simulink model "queueing"  (R2023b)
settings: Solver=VariableStepAuto  StartTime=0.0  StopTime=10.0  RelTol=1e-3
undefined symbols (not defined in the file or in its folder): m, n
settings Model: Creator=miha4  LastModifiedBy=RobotComp.ru
settings RTWCC: GPUComputeCapability=5.0

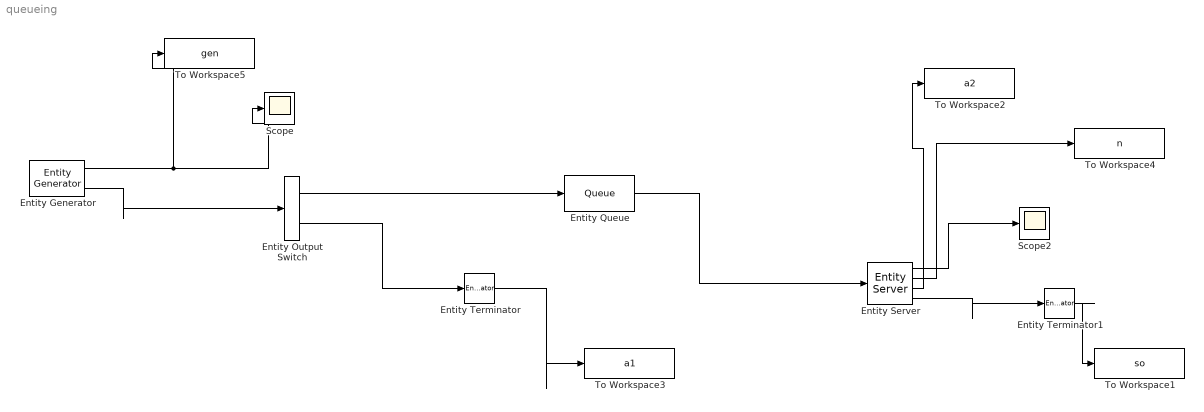
== system queueing ==
  Entity Output Switch : EntityOutputSwitch  InputPortMessageModes=m  OutputPortMessageModes=m,m  SwitchAttributeName=Attribute1
  Entity Generator : EntityGenerator  OutputPortMessageModes=n,m  TimeSource=MATLAB action  IntergenerationTimeAction=|  NumberEntitiesDeparted=on  EntityType=Structured  EntityTypeName=Entity
      | persistent rngInit;
      | if isempty(rngInit)
      |     seed = 12345;
      |     rng(seed);
      |     rngInit = true;
      | end
      | 
      | % Pattern: Exponential distribution
      | mu = 5;
      | dt = -mu * log(1 - rand());
      settings: OutputPortMap=o0,o3
  Entity Queue : Queue  InputPortMessageModes=m  OutputPortMessageModes=m  Capacity=4
  Entity Server : EntityServer  InputPortMessageModes=m  OutputPortMessageModes=n,n,n,m  Capacity=c  ServiceTimeSource=MATLAB action  ServiceTimeValue=500  ServiceTimeAction=|  NumberEntitiesDeparted=on  NumberEntitiesInBlock=on  Utilization=on
      | persistent rngInit;
      | if isempty(rngInit)
      |     seed = 12345;
      |     rng(seed);
      |     rngInit = true;
      | end
      | 
      | % Pattern: Uniform distribution
      | % m: Minimum, M: Maximum
      | m = 2; M = 5;
      | dt = m + (M - m) * rand;
      settings: OutputPortMap=o0,o1,o5,o9
  Entity Terminator : EntityTerminator  InputPortMessageModes=m  NumberEntitiesArrived=on
      settings: OutputPortMap=o0
  Entity Terminator1 : EntityTerminator  InputPortMessageModes=m  NumberEntitiesArrived=on
      settings: OutputPortMap=o0
  Scope : Scope
  Scope2 : Scope
  To Workspace1 : ToWorkspace  VariableName=so  SaveFormat=Timeseries  SampleTime=-1
  To Workspace2 : ToWorkspace  VariableName=a2  SaveFormat=Timeseries  SampleTime=-1
  To Workspace3 : ToWorkspace  VariableName=a1  SaveFormat=Timeseries  SampleTime=-1
  To Workspace4 : ToWorkspace  VariableName=n  SaveFormat=Timeseries  SampleTime=-1
  To Workspace5 : ToWorkspace  VariableName=gen  SaveFormat=Timeseries  SampleTime=-1
  wires:
  Entity Output Switch/1 -> Entity Queue/1
  Entity Server/3 -> To Workspace2/1
  Entity Output Switch/2 -> Entity Terminator/1
  Entity Generator/2 -> Entity Output Switch/1
  Entity Terminator/1 -> To Workspace3/1
  Entity Server/1 -> Scope2/1
  Entity Generator/1 -> To Workspace5/1, Scope/1
  Entity Server/2 -> To Workspace4/1
  Entity Terminator1/1 -> To Workspace1/1
  Entity Server/4 -> Entity Terminator1/1
  Entity Queue/1 -> Entity Server/1
